simulink library "eclipseCheck"  (R2018b)
settings: Solver=VariableStepAuto  StartTime=0.0  StopTime=10.0  RelTol=1e-3
settings Model: Creator=devantormey  LastModifiedBy=taylorreynolds

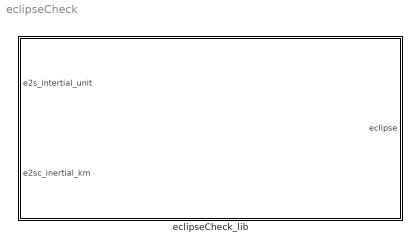
== system eclipseCheck ==
  eclipseCheck_lib : Subsystem

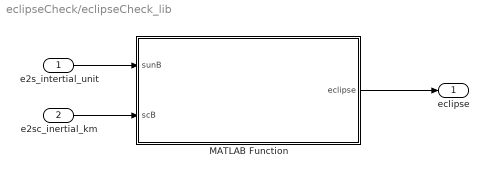
== system eclipseCheck/eclipseCheck_lib ==
  e2s_intertial_unit : Inport
  e2sc_inertial_km : Inport  Port=2
  MATLAB Function : MATLAB Function  TreatAsAtomicUnit=on
  eclipse : Outport
  wires:
  e2s_intertial_unit/1 -> MATLAB Function/1(sunB)
  e2sc_inertial_km/1 -> MATLAB Function/2(scB)
  MATLAB Function/1(eclipse) -> eclipse/1

== matlab function eclipseCheck/eclipseCheck_lib/MATLAB Function ==
  data: sunB input; eclipse output boolean; scB input; simParams parameter
function eclipse = fcn(sunB,scB,simParams)
%#codegen
% DESCRIPTION
% ~~~~~~~~~~~~~
% This function computes the mean longitude phi_s and mean anomoly M_s of
% the sun from an incoming time stampe Tut1. Tut1 is computed using the
% BLANK formula
% ~~~~~~~~~~~~~~~~~~~~~~~~~~~~~~~~~~~~~~
% Variables
% sunI      - this is the sun from the inertial frame
% scI       - this is the spacecraft position from inertial frame
% eclipse   - will be a true/false if we are in/out of eclipse [boolean]
% Re        - is the earth radius
% AU2Km     - convert from AU to km
% ~~~~~~~~~~~~~~~~~~~~~~~~~~~~~~~~~~~~~~
light = false;

Re      = simParams.constants.global.r_earth_km;
AU2Km   = simParams.constants.convert.AU2KM;

sunB = sunB*AU2Km; 

tmin = ( norm(scB)^2 - dot(scB,sunB) )/ ( norm(scB)^2 +  norm(sunB)^2 - 2*(dot(scB,sunB)) );

if (tmin < 0) || (tmin > 1)
    light = true;
end
if (1 - tmin)*norm(scB)^2 + dot(scB,sunB)*tmin >= 1.0 * Re.^2
    light = true;
end

if (light)
    eclipse = false;
else
    eclipse = true;
end

end
